simulink model "Practica7seminario"  (R2017b)
settings: Solver=VariableStepAuto  StartTime=0.0  StopTime=5  RelTol=1e-3
values from neighbouring files (symbols this model uses):
  C1 = 1e-6    (= 1e-06)    [PR7.m]
  C2 = 1e-6    (= 1e-06)    [PR7.m]
  R1 = 5e6    (= 5000000)    [PR7.m]
  R2 = 5e6    (= 5000000)    [PR7.m]
  R3 = 5e6    (= 5000000)    [PR7.m]
settings Model: Creator=Charles  LastModifiedBy=Charles

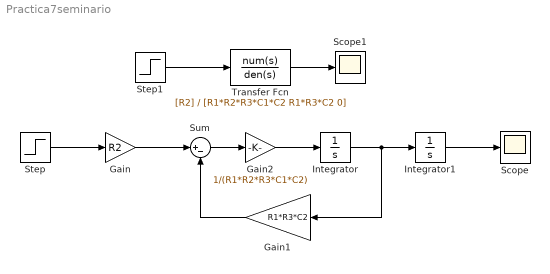
== system Practica7seminario ==
  Gain : Gain  Gain=R2
  Gain1 : Gain  Gain=R1*R3*C2
  Gain2 : Gain  Gain=1/(R1*R2*R3*C1*C2)
  Integrator : Integrator
  Integrator1 : Integrator
  Scope : Scope
  Scope1 : Scope
  Step : Step  Time=0  After=5  SampleTime=0
  Step1 : Step  Time=0  After=5  SampleTime=0
  Sum : Sum  Inputs=|+-
  Transfer Fcn : TransferFcn  Numerator=[R2]  Denominator=[R1*R2*R3*C1*C2 R1*R3*C2 0]
  wires:
  Step/1 -> Gain/1
  Gain/1 -> Sum/1
  Integrator/1 -> Gain1/1, Integrator1/1
  Integrator1/1 -> Scope/1
  Gain1/1 -> Sum/2
  Sum/1 -> Gain2/1
  Gain2/1 -> Integrator/1
  Step1/1 -> Transfer Fcn/1
  Transfer Fcn/1 -> Scope1/1
